simulink model "output_X"  (R2019b)
settings: Solver=ode45  StartTime=0.0  StopTime=10.0  MaxStep=0.2  RelTol=1e-3
settings Model: Creator=kaba  LastModifiedBy=kaba
settings DataIOCC: ExternalInput=[t, u1, u2]  LoadExternalInput=on  SaveFormat=Array  SignalLogging=off  DSMLogging=off

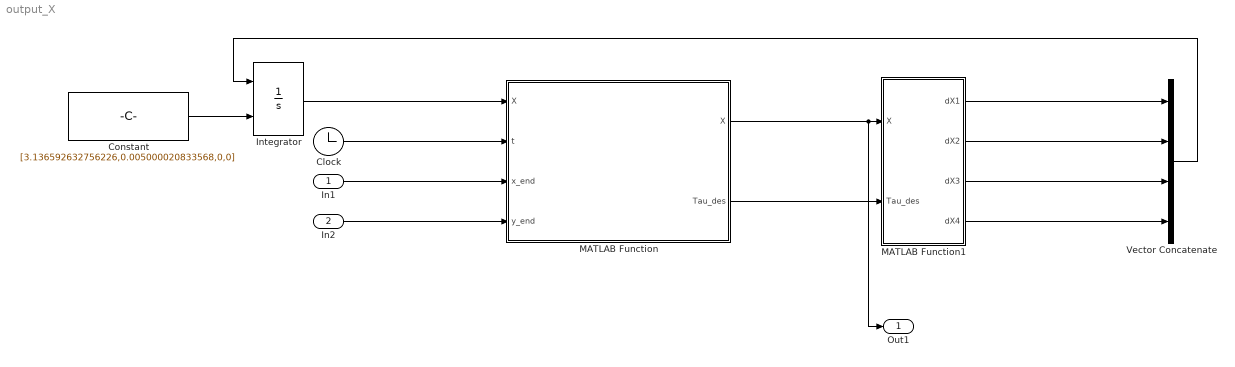
== system output_X ==
  In1 : Inport
  In2 : Inport  Port=2
  Clock : Clock
  Constant : Constant  Value=[3.136592632756226,0.005000020833568,0,0]
  Integrator : Integrator  InitialConditionSource=external
  MATLAB Function : MATLAB Function  TreatAsAtomicUnit=on
  MATLAB Function1 : MATLAB Function  TreatAsAtomicUnit=on
  Vector Concatenate : Concatenate  NumInputs=4
  Out1 : Outport
  wires:
  Constant/1 -> Integrator/2
  Integrator/1 -> MATLAB Function/1("X ")
  Vector Concatenate/1 -> Integrator/1
  MATLAB Function/1(X) -> Out1/1, MATLAB Function1/1(X)
  MATLAB Function1/2(dX2) -> Vector Concatenate/2
  In2/1 -> MATLAB Function/4(y_end)
  In1/1 -> MATLAB Function/3(x_end)
  MATLAB Function1/3(dX3) -> Vector Concatenate/3
  MATLAB Function/2(Tau_des) -> MATLAB Function1/2(Tau_des)
  MATLAB Function1/4(dX4) -> Vector Concatenate/4
  Clock/1 -> MATLAB Function/2(t)
  MATLAB Function1/1(dX1) -> Vector Concatenate/1

== matlab function output_X/MATLAB Function1 ==
  data: X input; dX1 output; Tau_des input; dX2 output; dX3 output; dX4 output
function [dX1,dX2,dX3,dX4] = solve_dX(X,Tau_des)

    %% INPUT PARAMETERS
    l1= 1 ;% (m)Length of element 1
    lc1= 0.5 ;%(m) Distance of CM of element 1 from source end
    m1= 6;% (kg) Mass of element 1
    j1= 2;% (kg-m^2) Moment of Inertia of element 1 about its CM

    lc2= 0.5;% (m)Distance of CM of element 2 from source end
    m2= 6;% (kg) Mass of element 2
    j2= 2;% (kg-m^2)Moment of Inertia of element 2 about its CM

    g= 0; % (m/sec^2) Acceleration due to gravity
    
    th1=X(1);
    th2=X(2);
    th1d=X(3);
    th2d=X(4);
    
    %% Simulation Data
    c1=cos(th1);
    c2=cos(th2);
    c21=cos(th2-th1);
    s21=sin(th2-th1);
    
    %%%%%% Dynamic control matrices
    M = [ j1+m2*l1^2, m2*l1*lc2*c21;
          m2*l1*lc2*c21, j2+m2*lc2^2];
    V = [0, -m2*l1*lc2*s21;
        m2*l1*lc2*s21, 0];
    G = [m1*g*lc1*c1+m2*g*l1*c1;
        m2*g*lc2*c2];
    %%%%%%%%%%%%%%%%%%%%%%%%%
    
    %% Generating differential
    [THDD]=M\(Tau_des- V*[th1d^2;th2d^2]-G); %%% Deriving angular acc

    %% Simulation Update
    dX1= th1d;
    dX2= th2d;
    dX3= THDD(1);
    dX4= THDD(2);

== matlab function output_X/MATLAB Function ==
  data: X input; X output; t input; Tau_des output; x_end input; y_end input

function [X,Tau_des] = solve_tau_des(X,t,x_end,y_end)

    %% INPUT PARAMETERS
    l1= 1 ;% (m)Length of element 1
    lc1= 0.5 ;%(m) Distance of CM of element 1 from source end
    m1= 6;% (kg) Mass of element 1
    j1= 2;% (kg-m^2) Moment of Inertia of element 1 about its CM

    lc2= 0.5;% (m)Distance of CM of element 2 from source end
    m2= 6;% (kg) Mass of element 2
    j2= 2;% (kg-m^2)Moment of Inertia of element 2 about its CM

    g= 0; % (m/sec^2) Acceleration due to gravity
    Kp1= [100, 0;0, 100];
    Kd1= [20, 0;0, 20];
        
    
    th1=X(1);
    th2=X(2);
    th1d=X(3);
    th2d=X(4);
    
    
    %% CREATING IMPORTANT MATRICES IN THE GOVERNING EQUATION
    
    %% Acquiring desired theta values for points exactly on the ellipse%%%%%%%
    THETA_DES=TH_DES_INFO(t,[th1,th2],x_end,y_end);
    th1_des=THETA_DES(1);
    th2_des=THETA_DES(2);
    th1d_des=THETA_DES(3);
    th2d_des=THETA_DES(4);
    th1dd_des=THETA_DES(5);
    th2dd_des=THETA_DES(6);
    
    c1_des=cos(th1_des);
    c2_des=cos(th2_des);
    c21_des=cos(th2_des-th1_des);
    s21_des=sin(th2_des-th1_des);
    
    %% Dynamic control matrices : Desired
    Mdes = [ j1+m2*l1^2, m2*l1*lc2*c21_des;
          m2*l1*lc2*c21_des, j2+m2*lc2^2];
    Vdes = [0, -m2*l1*lc2*s21_des;
        m2*l1*lc2*s21_des, 0];
    Gdes = [m1*g*lc1*c1_des+m2*g*l1*c1_des;
        m2*g*lc2*c2_des];
    
    %% Control Torque (based on ideal situation)
    % Tau_des1= Mdes*[th1dd_des;th2dd_des] + Vdes*[th1d_des^2;th2d_des^2]+Gdes; %% Control Torque
    Tau_des= Gdes+ Vdes*[th1d_des^2;th2d_des^2] + Mdes*( [th1dd_des;th2dd_des] + Kp1*([th1_des;th2_des]-[th1;th2]) + Kd1*([th1d_des;th2d_des]-[th1d;th2d])); %% Control Torque
